simulink model "DEA_strip_t6_triangle"  (R2018a)
settings: Solver=VariableStepAuto  StartTime=0.0  StopTime=param_simtime  MaxStep=0.001  EnableMultiTasking=on
InitFcn:
  | Parameter;
values from neighbouring files (symbols this model uses):
  param_f_res = 34.5    [plot_task6.m]
  param_g = 9.81    [plot_task6.m]
  param_k1 = 10800    [plot_task6.m]
  param_k2 = 43200    [plot_task6.m]
  param_l1 = 0.0164    [plot_task6.m]
  param_m1 = 0.25    [plot_task6.m]
  param_m2 = 0.25    [plot_task6.m]
  param_N = 8    [plot_task6.m]
  param_y2 = -1.135*10^-4    (= -0.0001135)    [plot_task6.m]
  param_ys0 = 0.02    [plot_task6.m]
libraries: simulink x3, dspxfrm3 x2
settings Model: Creator=Johannes  LastModifiedBy=Tim
settings DataIOCC: LimitDataPoints=on  SaveFormat=Array  SignalLoggingSaveFormat=ModelDataLogs
settings OptimizationCC: LifeSpan=inf
settings DebuggingCC: UnderspecifiedInitializationDetection=Classic  MergeDetectMultiDrivingBlocksExec=none  SolverPrmCheckMsg=warning  MultiTaskDSMMsg=warning  MultiTaskCondExecSysMsg=none  SFUnexpectedBacktrackingDiag=warning  SFNoUnconditionalDefaultTransitionDiag=warning  SFExecutionAtInitializationDiag=none
settings HardwareCC: ProdBitPerPointer=32  ProdBitPerSizeT=32  ProdBitPerPtrDiffT=32  ProdLargestAtomicFloat=None  ProdIntDivRoundTo=Undefined  ProdEndianess=Unspecified  ProdWordSize=32  ProdHWDeviceType=32-bit Generic
settings ModelReferenceCC: PropagateSignalLabelsOutOfModel=off
settings CodeAppCC: StateflowObjectComments=on
settings GRTTargetCC: TargetLangStandard=C89/C90 (ANSI)  GeneratePreprocessorConditionals=Disable all
settings ConfigComp: CovMetricSettings=dw  CovHtmlReporting=on  CovSaveCumulativeToWorkspaceVar=on  CovSaveSingleToWorkspaceVar=on  CovExternalEMLEnable=off

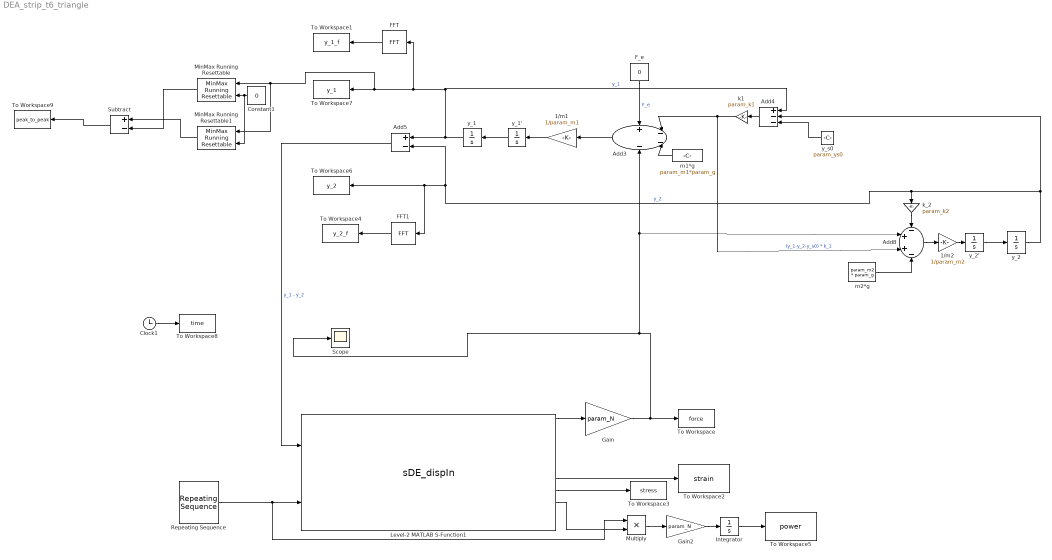
== system DEA_strip_t6_triangle ==
  1/m1 : Gain  Gain=1/param_m1
  "1/m2 " : Gain  Gain=1/param_m2
  Add3 : Sum  Inputs=+---
  Add4 : Sum  Inputs=+--
  Add5 : Sum  Inputs=+-
  Add8 : Sum  Inputs=-++-
  Clock1 : Clock
  Constant1 : Constant  Value=0
  FFT : dspxfrm3/FFT  FFTImplementation=Auto  CompMethod=Table lookup  TableOpt=NEW  TableOptActive=Speed  BitRevOrder=off  Normalize=off  InheritFFTLength=on  FFTLength=64  WrapInput=on  roundingMode=Floor  overflowMode=off  firstCoeffDataTypeStr=Inherit: Same word length as input  firstCoeffLastDataTypeStr=Inherit: Same word length as input  outputMin=[]  outputMax=[]
  FFT1 : dspxfrm3/FFT  FFTImplementation=Auto  CompMethod=Table lookup  TableOpt=NEW  TableOptActive=Speed  BitRevOrder=off  Normalize=off  InheritFFTLength=on  FFTLength=64  WrapInput=on  roundingMode=Floor  overflowMode=off  firstCoeffDataTypeStr=Inherit: Same word length as input  firstCoeffLastDataTypeStr=Inherit: Same word length as input  outputMin=[]  outputMax=[]
  "F_e " : Constant  Value=0
  Gain : Gain  Gain=param_N
  Gain2 : Gain  Gain=param_N
  Integrator : Integrator
  Level-2 MATLAB S-Function1 : M-S-Function  FunctionName=sDE_dispIn  Parameters=params, initConds
      mask Display:
      | color('black');
      | patch(4*[-1 1 1 -1],1.75*[-1 -1 1 1],[1 1 1]);
      | patch(2*[-1 1 1 -1],1.2*[-1 -1 1 1],[0 0 0]);
      | patch(1.95*[-1 1 1 -1],0.8*[-1 -1 1 1],[1 1 1]);
      | disp('DE Actuator');
      | 
      | color('blue');
      | port_label('input', 1, 'l_1 [m]','texmode','on');
      | port_label('input', 2, 'v [V]','texmode','on');
      | 
      | color('red');
      | port_label('output', 1, 'F_1 [N]','texmode','on');
      | port_label('output', 2, 'x_{v1} [-]','texmode','on');
      | port_label('output', 3, 'x_{v2} [-]','texmode','on');
      | port_label('output', 4, '\epsilon_2 [-]','texmode','on');
      | port_label('output', 5, 'q [C]','texmode','on');
      | port_label('output', 6, '\epsilon_1 [-]','texmode','on');
      | port_label('output', 7, '\sigma_1 [Pa]','texmode','on');
      | port_label('output', 8, 'i [A]','texmode','on');
      | port_label('output', 9, 'v_{DE} [V]','texmode','on');
      | port_label('output', 10, 'C [F]','texmode','on');
  MinMax Running Resettable : simulink/Math Operations/MinMax Running Resettable  Function=min  vinit=0
  MinMax Running Resettable1 : simulink/Math Operations/MinMax Running Resettable  Function=max  vinit=0
  Multiply : Product
  Repeating Sequence : simulink/Sources/Repeating Sequence  rep_seq_t=[0 (1/(2*param_f_res)) 1/param_f_res]  rep_seq_y=[0 2500 0]
  Scope : Scope
  Subtract : Sum  Inputs=+-
  To Workspace : ToWorkspace  VariableName=force  SampleTime=-1
  To Workspace1 : ToWorkspace  VariableName=y_1_f  SampleTime=-1
  To Workspace2 : ToWorkspace  VariableName=strain  SampleTime=-1
  To Workspace3 : ToWorkspace  VariableName=stress  SampleTime=-1
  To Workspace4 : ToWorkspace  VariableName=y_2_f  SampleTime=-1
  To Workspace5 : ToWorkspace  VariableName=power  SampleTime=-1
  To Workspace6 : ToWorkspace  VariableName=y_2  SampleTime=-1
  To Workspace7 : ToWorkspace  VariableName=y_1  SampleTime=-1
  To Workspace8 : ToWorkspace  VariableName=time  SampleTime=-1
  To Workspace9 : ToWorkspace  VariableName=peak_to_peak  SampleTime=-1
  k1 : Gain  Gain=param_k1
  k_2 : Gain  Gain=param_k2
  m1*g : Constant  Value=param_m1*param_g
  m2*g : Constant  Value=param_m2 * param_g
  y_1 : Integrator  InitialCondition=param_y2 + param_l1
  y_1' : Integrator
  y_2 : Integrator  InitialCondition=param_y2
  y_2' : Integrator
  y_s0 : Constant  Value=param_ys0
  wires:
  Level-2 MATLAB S-Function1/1 -> Gain/1
  Level-2 MATLAB S-Function1/6 -> To Workspace2/1
  Level-2 MATLAB S-Function1/7 -> To Workspace3/1
  Gain/1 -> Scope/1, Add3/4, Add8/2, To Workspace/1
  m1*g/1 -> Add3/3
  y_s0/1 -> Add4/3
  Add3/1 -> 1/m1/1
  1/m1/1 -> y_1'/1
  y_1'/1 -> y_1/1
  y_1/1 -> FFT/1, MinMax Running Resettable1/1, MinMax Running Resettable/1, To Workspace7/1, Add4/1, Add5/1  "y_1"
  y_2/1 -> k_2/1, Add5/2, FFT1/1, To Workspace6/1, Add4/2  "y_2"
  Add5/1 -> Level-2 MATLAB S-Function1/1  "y_1 - y_2"
  Add4/1 -> k1/1
  k1/1 -> Add8/3, Add3/2  "(y_1-y_2-y_s0) * k_1"
  m2*g/1 -> Add8/4
  y_2'/1 -> y_2/1
  Add8/1 -> "1/m2 "/1
  "1/m2 "/1 -> y_2'/1
  "F_e "/1 -> Add3/1  "F_e"
  k_2/1 -> Add8/1
  Clock1/1 -> To Workspace8/1
  FFT/1 -> To Workspace1/1
  FFT1/1 -> To Workspace4/1
  Level-2 MATLAB S-Function1/8 -> Multiply/2
  Multiply/1 -> Gain2/1
  Gain2/1 -> Integrator/1
  Integrator/1 -> To Workspace5/1
  Constant1/1 -> MinMax Running Resettable1/2, MinMax Running Resettable/2
  MinMax Running Resettable/1 -> Subtract/2
  MinMax Running Resettable1/1 -> Subtract/1
  Subtract/1 -> To Workspace9/1
  Repeating Sequence/1 -> Multiply/1, Level-2 MATLAB S-Function1/2
